simulink model "benchmark_model"  (R2021a)
settings: Solver=ode1  StartTime=0.0  StopTime=Tend  FixedStep=0.0001  MaxStep=0.1  MinStep=0.0001  AbsTol=0.01  EnableMultiTasking=on
undefined symbols (not defined in the file): A1, A2, AL, AM0, AREA, BORE, C_EGR, c_f, c_T, CAIR, cCO, cCO2, cH2, cH2O, cHC, cN2, CO, CO2, cO2, DEN0, DiscIntNeverNeededParam, EGR_dia, EGR_sk, EX_AREA, EX_M_AR, EXO, FD0, FOM, FR0, FR_C1, FR_C2, FR_C3, FR_C4, FR_C5, H2, H2O, HC, INC, INO, KET, Kex, Kh, MAS0, MCh, MHC, MN2, MO2, MOLcylT, N2, O2, PR0, R150, Rabs, SPEC, TBORE, Th_HC, Th_knock, THEX, THIN, TM0 ... (+9)
libraries: pid_lib x1
(part 3 of 6)

== system benchmark_model/ENGINE/engine_s/cylinders/cyl2/cyl/cyl_conc ==
  mol_bs : Inport
  mol_us : Inport  Port=2
  Add : Sum
  Divide : Product  Inputs=*/
  Sum of Elements : Sum  Inputs=+
  cyl_conc : Outport  PortDimensions=7
  mix_mol : Outport  Port=2  PortDimensions=7
  wires:
  Divide/1 -> cyl_conc/1
  mol_bs/1 -> Add/1
  mol_us/1 -> Add/2
  Sum of Elements/1 -> Divide/2
  Add/1 -> mix_mol/1, Divide/1, Sum of Elements/1

== system benchmark_model/ENGINE/engine_s/cylinders/cyl2/cyl/frame ==
  rps : Inport
  rad : Inport  Port=2
  VT : Inport  Port=3
  SA : Inport  Port=4
  tr_inc : Inport  Port=5
  mol_s : Inport  Port=6
  AF : Inport  Port=7
  KL : Inport  Port=8
  EGR : Inport  Port=9
  Init_cyl_gas : Subsystem
  Product : Product  RndMeth=Zero
  Product1 : Product  RndMeth=Zero
  Product2 : Product  RndMeth=Zero
  ratio_burnt1 : Subsystem
  burning gas : Outport
  q : Outport  Port=2
  burnt_gas : Outport  Port=3
  QR : Outport  Port=4
  QA : Outport  Port=5
  af : Outport  Port=6
  Qmax : Outport  Port=7
  wires:
  VT/1 -> ratio_burnt1/7(VT)
  ratio_burnt1/3(Q) -> QA/1
  EGR/1 -> ratio_burnt1/6(EGR)
  ratio_burnt1/2(QR) -> QR/1
  SA/1 -> ratio_burnt1/5(SA)
  KL/1 -> ratio_burnt1/4(KL)
  AF/1 -> ratio_burnt1/3(AF)
  tr_inc/1 -> Init_cyl_gas/1(tr_inc)
  mol_s/1 -> Init_cyl_gas/2(mol_s)
  Init_cyl_gas/4(af) -> af/1
  rad/1 -> ratio_burnt1/2(rad)
  rps/1 -> ratio_burnt1/1(rps)
  ratio_burnt1/1(burnt_ratio) -> Product1/1, Product2/1, Product/1
  Init_cyl_gas/2(Qmax) -> Product1/2, Qmax/1
  Product/1 -> burning gas/1
  Init_cyl_gas/1(init_gas) -> Product/2
  Product1/1 -> q/1
  Product2/1 -> burnt_gas/1
  Init_cyl_gas/3(b_comp) -> Product2/2

== system benchmark_model/ENGINE/engine_s/cylinders/cyl2/cyl/heat_trans ==
  rps : Inport
  pc : Inport  Port=2
  tc : Inport  Port=3
  vol : Inport  Port=4
  Constant5 : Constant  Value=TW0
  Gain : Gain  Gain=Kh
  Product : Product  RndMeth=Zero
  cal_cyl_ar : Subsystem
  cal_qw : Subsystem
  cyl_wall : Subsystem
  qw : Outport
  wires:
  Gain/1 -> qw/1, cyl_wall/1(qw_v)
  cal_cyl_ar/1(cyl_ar) -> Product/1
  vol/1 -> cal_cyl_ar/1(vol)
  Constant5/1 -> cyl_wall/2(Tw0)
  Product/1 -> Gain/1
  cal_qw/1(qw) -> Product/2
  cyl_wall/1(Tw) -> cal_qw/4(Tw)
  tc/1 -> cal_qw/3(Tg)
  rps/1 -> cal_qw/2(rps)
  pc/1 -> cal_qw/1(pc)

== system benchmark_model/ENGINE/engine_s/cylinders/cyl2/cyl/knock_Integral ==
  pc : Inport
  Tc : Inport  Port=2
  Qmax : Inport  Port=3
  rad : Inport  Port=4
  rps : Inport  Port=5
  QA : Inport  Port=6
  Constant : Constant
  Constant1 : Constant  Value=(180-EXO-3)*pi/180
  Constant2 : Constant
  Logical Operator : Logic  Operator=OR  AllPortsSameDT=off  OutDataTypeStr=boolean
  Product : Product
  Relational Operator : RelationalOperator  OutDataTypeStr=boolean  RndMeth=Nearest
  Relational Operator1 : RelationalOperator  OutDataTypeStr=boolean  RndMeth=Nearest
  Subsystem1 : Subsystem
  Switch : Switch  Threshold=0.5
  Triggered Subsystem : Subsystem  TreatAsAtomicUnit=on
  ki : Outport
  ki1 : Outport  Port=2
  wires:
  Triggered Subsystem/1(AI_Q) -> Product/1
  Constant2/1 -> Switch/3
  Switch/1 -> Triggered Subsystem/1(QA_max)
  Logical Operator/1 -> Triggered Subsystem/Trigger
  Relational Operator1/1 -> Logical Operator/2, Switch/2
  Relational Operator/1 -> Logical Operator/1
  QA/1 -> Triggered Subsystem/2(QA), Switch/1
  Qmax/1 -> Product/2
  Product/1 -> ki1/1
  Constant1/1 -> Relational Operator1/2
  Constant/1 -> Relational Operator/2
  Subsystem1/1(ki) -> ki/1, Relational Operator/1
  rad/1 -> Subsystem1/4(rad), Relational Operator1/1
  Tc/1 -> Subsystem1/3(Tc)
  rps/1 -> Subsystem1/2(rps)
  pc/1 -> Subsystem1/1(pc)

== system benchmark_model/ENGINE/engine_s/cylinders/cyl2/cyl/ramining ratio of fuel ==
  rad : Inport
  QA : Inport  Port=2
  Constant1 : Constant  Value=(180-EXO-3)*pi/180
  Memory : Memory
  Relational Operator1 : RelationalOperator  OutDataTypeStr=boolean  RndMeth=Nearest
  Triggered Subsystem : Subsystem  TreatAsAtomicUnit=on
  r_HC : Outport
  wires:
  Memory/1 -> Triggered Subsystem/1(QA)
  Relational Operator1/1 -> Triggered Subsystem/Trigger
  rad/1 -> Relational Operator1/1
  QA/1 -> Memory/1
  Triggered Subsystem/1(AI_Q) -> r_HC/1
  Constant1/1 -> Relational Operator1/2

== system benchmark_model/ENGINE/engine_s/cylinders/cyl2/cyl/unburnt_gass ==
  Nfuel : Inport
  burning : Inport  Port=2
  gas_in : Inport  Port=3
  gas_out : Inport  Port=4
  trig_mix : Inport  Port=5
  mix_mol : Inport  Port=6
  Mass_Int : Integrator  ExternalReset=rising  InitialConditionSource=external  InitialCondition=MAS0
  Memory1 : Memory
  Memory2 : Memory
  Sum : Sum  Inputs=+--  InputSameDT=on  SaturateOnIntegerOverflow=on  OutDataTypeStr=Inherit: Same as first input
  add_fuel1 : Subsystem
  init&trig : Subsystem  mask{NHC=cHC*MOLcylT, NCO2=cCO2*MOLcylT, NCO=cCO*MOLcylT, NO2=cO2*MOLcylT, NH2=cH2*MOLcylT, NH2O=cH2O*MOLcylT, NN2=cN2*MOLcylT}
      mask prompts: NHC "initial HC mol"; NCO2 "initial CO2 mol"; NCO "initial CO mol"; NO2 "initial O2 mol"; NH2 "initial H2 mol"; NH2O "initial H2O mol"; NN2 "initial N2 mol"
  mol_us : Outport  InitialOutput=0
  wires:
  Memory1/1 -> init&trig/2(value)
  trig_mix/1 -> Memory2/1
  Memory2/1 -> Mass_Int/2, init&trig/1(trig)
  add_fuel1/1(add_fuel) -> Sum/1
  Nfuel/1 -> add_fuel1/1(Nfuel)
  gas_in/1 -> add_fuel1/2(mol)
  init&trig/1(init) -> Mass_Int/3
  mix_mol/1 -> Memory1/1
  Mass_Int/1 -> mol_us/1
  burning/1 -> Sum/3
  Sum/1 -> Mass_Int/1
  gas_out/1 -> Sum/2

== system benchmark_model/ENGINE/engine_s/cylinders/cyl2/selectors/Triggered Subsystem1 ==
  sa : Inport
  Trigger : TriggerPort  VariantControl=(inherit)
  req_sa : Outport  InitialOutput=[20]
  wires:
  sa/1 -> req_sa/1

== system benchmark_model/ENGINE/engine_s/cylinders/cyl2/selectors/Triggered Subsystem2 ==
  int_mc : Inport
  Trigger : TriggerPort  VariantControl=(inherit)
  O2_mol : Outport  InitialOutput=[1.0e-19]
  wires:
  int_mc/1 -> O2_mol/1

== system benchmark_model/ENGINE/engine_s/cylinders/cyl2/selectors/Triggered Subsystem3 ==
  int_mc : Inport
  Trigger : TriggerPort  VariantControl=(inherit)
  MC : Outport  InitialOutput=[1.0e-19]
  wires:
  int_mc/1 -> MC/1

== system benchmark_model/ENGINE/engine_s/cylinders/cyl2/selectors/effective_O2_flow ==
  fml : Inport
  Gain : Gain  Gain=1+y/4
  Gain1 : Gain  Gain=0.5
  Gain2 : Gain  Gain=0.5
  Selector : Selector  InputPortWidth=7  IndexOptions=Index vector (dialog)  Indices=[4]  OutputSizes=1
  Selector1 : Selector  InputPortWidth=7  IndexOptions=Index vector (dialog)  Indices=[1]  OutputSizes=1
  Selector2 : Selector  InputPortWidth=7  IndexOptions=Index vector (dialog)  Indices=[3]  OutputSizes=1
  Selector3 : Selector  InputPortWidth=7  IndexOptions=Index vector (dialog)  Indices=[5]  OutputSizes=1
  Subtract : Sum  Inputs=+---
  fO2_mol : Outport
  wires:
  Gain2/1 -> Subtract/4
  Gain1/1 -> Subtract/3
  Selector3/1 -> Gain2/1
  Selector2/1 -> Gain1/1
  Gain/1 -> Subtract/2
  Selector1/1 -> Gain/1
  Selector/1 -> Subtract/1
  fml/1 -> Selector3/1, Selector2/1, Selector1/1, Selector/1
  Subtract/1 -> fO2_mol/1

== system benchmark_model/ENGINE/engine_s/cylinders/cyl2/selectors/fuel_behavior ==
  MC : Inport
  fi : Inport  Port=2
  rps : Inport  Port=3
  Trigger : TriggerPort  VariantControl=(inherit)
  Discrete-Time Integrator : DiscreteIntegrator  SampleTime=-1  ICPrevOutput=DiscIntNeverNeededParam  ICPrevScaledInput=DiscIntNeverNeededParam
  Terminator : Terminator
  Terminator3 : Terminator
  fc : Outport  InitialOutput=[0]
  sum_fc : Outport  Port=2  InitialOutput=[0]
  wires:
  Discrete-Time Integrator/1 -> sum_fc/1
  rps/1 -> Terminator/1
  MC/1 -> Terminator3/1
  fi/1 -> fc/1, Discrete-Time Integrator/1

== system benchmark_model/ENGINE/engine_s/cylinders/cyl2/selectors/selector ==
  st : Inport
  ECU_sa : Inport  Port=2
  ECU_fi : Inport  Port=3
  Saturation : Saturate  UpperLimit=inf  LowerLimit=0
  Selector : Selector  InputPortWidth=4  IndexOptions=Index vector (dialog)  Indices=[2]  OutputSizes=[(-2)]
  Selector2 : Selector  InputPortWidth=4  IndexOptions=Index vector (dialog)  Indices=[2]  OutputSizes=[(-2)]
  mod720(u,4*pi) : Subsystem
  rad : Outport
  sa : Outport  Port=2
  fi : Outport  Port=3
  wires:
  Selector2/1 -> sa/1
  ECU_fi/1 -> Saturation/1
  ECU_sa/1 -> Selector2/1
  st/1 -> Selector/1
  mod720(u,4*pi)/1(y) -> rad/1
  Saturation/1 -> fi/1
  Selector/1 -> mod720(u,4*pi)/1(u)

== system benchmark_model/ENGINE/engine_s/cylinders/cyl2/selectors/trig_MC ==
  deg : Inport
  ECU_vvt : Inport  Port=2
  Constant : Constant  Value=541+INC
  Gain : Gain  Gain=180/pi
  Relational Operator : RelationalOperator  OutDataTypeStr=boolean  RndMeth=Nearest
  Subtract : Sum
  flg_inc : Outport
  wires:
  Gain/1 -> Subtract/1
  Constant/1 -> Subtract/2
  ECU_vvt/1 -> Gain/1
  Subtract/1 -> Relational Operator/2
  Relational Operator/1 -> flg_inc/1
  deg/1 -> Relational Operator/1

== system benchmark_model/ENGINE/engine_s/cylinders/cyl2/selectors/trig_fi ==
  deg : Inport
  Constant : Constant  Value=361
  Relational Operator : RelationalOperator  OutDataTypeStr=boolean  RndMeth=Nearest
  flg_fi : Outport
  wires:
  Relational Operator/1 -> flg_fi/1
  deg/1 -> Relational Operator/1
  Constant/1 -> Relational Operator/2

== system benchmark_model/ENGINE/engine_s/cylinders/cyl2/selectors/trig_fi1 ==
  deg : Inport
  ECU_vvt : Inport  Port=2
  Constant : Constant  Value=360-INO-1
  Gain : Gain  Gain=180/pi
  Relational Operator : RelationalOperator  OutDataTypeStr=boolean  RndMeth=Nearest
  Subtract : Sum
  flg_fi : Outport
  wires:
  Constant/1 -> Subtract/2
  Subtract/1 -> Relational Operator/2
  Gain/1 -> Subtract/1
  ECU_vvt/1 -> Gain/1
  deg/1 -> Relational Operator/1
  Relational Operator/1 -> flg_fi/1

== system benchmark_model/ENGINE/engine_s/cylinders/cyl3/cyl/Energy_Int ==
  p : Inport
  qw : Inport  Port=2
  e_out : Inport  Port=3
  e_in : Inport  Port=4
  rad : Inport  Port=5
  rps : Inport  Port=6
  q : Inport  Port=7
  Constant : Constant  Value=PR0
  Product : Product  RndMeth=Zero
  Product1 : Product  RndMeth=Zero
  Subtract : Sum  Inputs=+-
  Sum2 : Sum  Inputs=+--+-  InputSameDT=on  SaturateOnIntegerOverflow=on  OutDataTypeStr=Inherit: Same as first input
  dvol : Subsystem
  int_e : Integrator  InitialCondition=(FD0/2.0)*PR0*VT
  int_pdv : Integrator
  E_mech : Outport  InitialOutput=0
  E : Outport  Port=2  InitialOutput=0
  wires:
  qw/1 -> Sum2/2
  e_out/1 -> Sum2/3
  Product/1 -> Sum2/5
  e_in/1 -> Sum2/4
  q/1 -> Sum2/1
  int_e/1 -> E/1
  Sum2/1 -> int_e/1
  rad/1 -> dvol/1(rad)
  dvol/1(dvol) -> Product1/1, Product/2
  rps/1 -> dvol/2(rps)
  int_pdv/1 -> E_mech/1
  p/1 -> Subtract/1, Product/1
  Constant/1 -> Subtract/2
  Subtract/1 -> Product1/2
  Product1/1 -> int_pdv/1

== system benchmark_model/ENGINE/engine_s/cylinders/cyl3/cyl/burnt_gass ==
  gas_in : Inport
  tr_mix : Inport  Port=2
  Mass_Int : Integrator  ExternalReset=rising  InitialCondition=[0;0;0;0;0;0;0]
  Memory2 : Memory
  mol_bs : Outport  PortDimensions=7  InitialOutput=0
  wires:
  Mass_Int/1 -> mol_bs/1
  gas_in/1 -> Mass_Int/1
  tr_mix/1 -> Memory2/1
  Memory2/1 -> Mass_Int/2

== system benchmark_model/ENGINE/engine_s/cylinders/cyl3/cyl/cal_cyl_state ==
  E : Inport
  mol_u : Inport  Port=2
  mol_b : Inport  Port=3
  rad : Inport  Port=4
  Add2 : Sum
  Constant : Constant  Value=SPEC
  Dot Product2 : DotProduct  InputSameDT=on  OutDataTypeStr=Inherit: Inherit via internal rule
  Dot Product3 : DotProduct  InputSameDT=on  OutDataTypeStr=Inherit: Inherit via internal rule
  Sum of Elements : Sum  Inputs=+
  cal_state : Subsystem
  cyl_vol : MATLAB Function  TreatAsAtomicUnit=on
  freedom : Constant  Value=FOM
  weight_mol : Constant  Value=WOM
  pc : Outport  InitialOutput=0
  tc : Outport  Port=2  InitialOutput=0
  vol : Outport  Port=3  InitialOutput=0
  cyl_st : Outport  Port=4  InitialOutput=0
  wires:
  E/1 -> cal_state/4(E)
  rad/1 -> cyl_vol/1(u)
  Constant/1 -> cyl_vol/2(SPEC)
  cal_state/1(pc) -> pc/1
  cal_state/2(tc) -> tc/1
  cal_state/3(cyl_st) -> cyl_st/1
  cyl_vol/1(vol) -> vol/1, cal_state/5(vol)
  weight_mol/1 -> Dot Product2/1
  mol_b/1 -> Add2/1
  mol_u/1 -> Add2/2
  Add2/1 -> Sum of Elements/1, Dot Product2/2, Dot Product3/1
  freedom/1 -> Dot Product3/2
  Sum of Elements/1 -> cal_state/2(n)
  Dot Product2/1 -> cal_state/1(m)
  Dot Product3/1 -> cal_state/3(f)

== system benchmark_model/ENGINE/engine_s/cylinders/cyl3/cyl/cal_torque ==
  E_mech : Inport
  Trigger : TriggerPort  VariantControl=(inherit)  PortDimensions=1
  Constant : Constant  Value=4*pi
  Divide : Product  Inputs=*/
  Subtract : Sum  Inputs=+-
  Unit Delay : UnitDelay  SampleTime=-1  HasFrameUpgradeWarning=on
  Torque : Outport
  wires:
  Unit Delay/1 -> Subtract/2
  E_mech/1 -> Subtract/1, Unit Delay/1
  Subtract/1 -> Divide/1
  Divide/1 -> Torque/1
  Constant/1 -> Divide/2

== system benchmark_model/ENGINE/engine_s/cylinders/cyl3/cyl/crank ==
  ecu : Inport
  Constant : Constant  Value=(180-EXO-1)*pi/180
  Constant2 : Constant  Value=(540+INC)*pi/180
  Relational Operator : RelationalOperator  OutDataTypeStr=boolean  RndMeth=Nearest
  Relational Operator2 : RelationalOperator  OutDataTypeStr=boolean  RndMeth=Nearest
  Selector : Selector  InputPortWidth=6  IndexOptions=Index vector (dialog)  Indices=1  OutputSizes=[(-2)]
  Selector1 : Selector  InputPortWidth=6  IndexOptions=Index vector (dialog)  Indices=[3]  OutputSizes=[(-2)]
  Selector2 : Selector  InputPortWidth=6  IndexOptions=Index vector (dialog)  Indices=[5]  OutputSizes=[(-2)]
  Selector3 : Selector  InputPortWidth=6  IndexOptions=Index vector (dialog)  Indices=2  OutputSizes=[(-2)]
  Selector4 : Selector  InputPortWidth=6  IndexOptions=Index vector (dialog)  Indices=6  OutputSizes=[(-2)]
  Selector5 : Selector  InputPortWidth=6  IndexOptions=Index vector (dialog)  Indices=6  OutputSizes=[(-2)]
  Subsystem1 : Subsystem
  Subtract : Sum  Inputs=+++
  inj_start : Subsystem
  mol_flow_rate : Subsystem
  trig_mix : Outport  PortDimensions=1
  rad : Outport  Port=2
  tr_inc : Outport  Port=3  PortDimensions=1
  SA : Outport  Port=4
  VT : Outport  Port=5
  Nfuel : Outport  Port=6
  wires:
  Selector/1 -> inj_start/1(rad), rad/1, Relational Operator2/1, Relational Operator/1
  Constant/1 -> Relational Operator/2
  ecu/1 -> Selector5/1, Selector4/1, Selector/1, Selector3/1, Selector2/1, Selector1/1
  Selector2/1 -> mol_flow_rate/1(rps)  "rps"
  Relational Operator2/1 -> tr_inc/1
  Selector3/1 -> SA/1
  Subtract/1 -> Relational Operator2/2
  Selector5/1 -> Subtract/1, VT/1
  Selector4/1 -> Subtract/3
  Constant2/1 -> Subtract/2
  Relational Operator/1 -> trig_mix/1
  inj_start/1(trig_inj) -> Subsystem1/1(trig_inj)
  Selector1/1 -> Subsystem1/2(fc)
  mol_flow_rate/1(N/s) -> Subsystem1/3(N/s)
  Subsystem1/1(N_fuel) -> Nfuel/1

== system benchmark_model/ENGINE/engine_s/cylinders/cyl3/cyl/cyl_conc ==
  mol_bs : Inport
  mol_us : Inport  Port=2
  Add : Sum
  Divide : Product  Inputs=*/
  Sum of Elements : Sum  Inputs=+
  cyl_conc : Outport  PortDimensions=7
  mix_mol : Outport  Port=2  PortDimensions=7
  wires:
  Add/1 -> Sum of Elements/1, Divide/1, mix_mol/1
  Sum of Elements/1 -> Divide/2
  mol_us/1 -> Add/2
  mol_bs/1 -> Add/1
  Divide/1 -> cyl_conc/1

== system benchmark_model/ENGINE/engine_s/cylinders/cyl3/cyl/frame ==
  rps : Inport
  rad : Inport  Port=2
  VT : Inport  Port=3
  SA : Inport  Port=4
  tr_inc : Inport  Port=5
  mol_s : Inport  Port=6
  AF : Inport  Port=7
  KL : Inport  Port=8
  EGR : Inport  Port=9
  Init_cyl_gas : Subsystem
  Product : Product  RndMeth=Zero
  Product1 : Product  RndMeth=Zero
  Product2 : Product  RndMeth=Zero
  ratio_burnt1 : Subsystem
  burning gas : Outport
  q : Outport  Port=2
  burnt_gas : Outport  Port=3
  QR : Outport  Port=4
  QA : Outport  Port=5
  af : Outport  Port=6
  Qmax : Outport  Port=7
  wires:
  Init_cyl_gas/3(b_comp) -> Product2/2
  Product2/1 -> burnt_gas/1
  Product1/1 -> q/1
  Init_cyl_gas/1(init_gas) -> Product/2
  Product/1 -> burning gas/1
  Init_cyl_gas/2(Qmax) -> Qmax/1, Product1/2
  ratio_burnt1/1(burnt_ratio) -> Product/1, Product2/1, Product1/1
  rps/1 -> ratio_burnt1/1(rps)
  rad/1 -> ratio_burnt1/2(rad)
  Init_cyl_gas/4(af) -> af/1
  mol_s/1 -> Init_cyl_gas/2(mol_s)
  tr_inc/1 -> Init_cyl_gas/1(tr_inc)
  AF/1 -> ratio_burnt1/3(AF)
  KL/1 -> ratio_burnt1/4(KL)
  SA/1 -> ratio_burnt1/5(SA)
  ratio_burnt1/2(QR) -> QR/1
  EGR/1 -> ratio_burnt1/6(EGR)
  ratio_burnt1/3(Q) -> QA/1
  VT/1 -> ratio_burnt1/7(VT)

== system benchmark_model/ENGINE/engine_s/cylinders/cyl3/cyl/heat_trans ==
  rps : Inport
  pc : Inport  Port=2
  tc : Inport  Port=3
  vol : Inport  Port=4
  Constant5 : Constant  Value=TW0
  Gain : Gain  Gain=Kh
  Product : Product  RndMeth=Zero
  cal_cyl_ar : Subsystem
  cal_qw : Subsystem
  cyl_wall : Subsystem
  qw : Outport
  wires:
  pc/1 -> cal_qw/1(pc)
  rps/1 -> cal_qw/2(rps)
  tc/1 -> cal_qw/3(Tg)
  cyl_wall/1(Tw) -> cal_qw/4(Tw)
  cal_qw/1(qw) -> Product/2
  Product/1 -> Gain/1
  Constant5/1 -> cyl_wall/2(Tw0)
  vol/1 -> cal_cyl_ar/1(vol)
  cal_cyl_ar/1(cyl_ar) -> Product/1
  Gain/1 -> cyl_wall/1(qw_v), qw/1

== system benchmark_model/ENGINE/engine_s/cylinders/cyl3/cyl/knock_Integral ==
  pc : Inport
  Tc : Inport  Port=2
  Qmax : Inport  Port=3
  rad : Inport  Port=4
  rps : Inport  Port=5
  QA : Inport  Port=6
  Constant : Constant
  Constant1 : Constant  Value=(180-EXO-3)*pi/180
  Constant2 : Constant
  Logical Operator : Logic  Operator=OR  AllPortsSameDT=off  OutDataTypeStr=boolean
  Product : Product
  Relational Operator : RelationalOperator  OutDataTypeStr=boolean  RndMeth=Nearest
  Relational Operator1 : RelationalOperator  OutDataTypeStr=boolean  RndMeth=Nearest
  Subsystem1 : Subsystem
  Switch : Switch  Threshold=0.5
  Triggered Subsystem : Subsystem  TreatAsAtomicUnit=on
  ki : Outport
  ki1 : Outport  Port=2
  wires:
  pc/1 -> Subsystem1/1(pc)
  rps/1 -> Subsystem1/2(rps)
  Tc/1 -> Subsystem1/3(Tc)
  rad/1 -> Relational Operator1/1, Subsystem1/4(rad)
  Subsystem1/1(ki) -> Relational Operator/1, ki/1
  Constant/1 -> Relational Operator/2
  Constant1/1 -> Relational Operator1/2
  Product/1 -> ki1/1
  Qmax/1 -> Product/2
  QA/1 -> Switch/1, Triggered Subsystem/2(QA)
  Relational Operator/1 -> Logical Operator/1
  Relational Operator1/1 -> Switch/2, Logical Operator/2
  Logical Operator/1 -> Triggered Subsystem/Trigger
  Switch/1 -> Triggered Subsystem/1(QA_max)
  Constant2/1 -> Switch/3
  Triggered Subsystem/1(AI_Q) -> Product/1

== system benchmark_model/ENGINE/engine_s/cylinders/cyl3/cyl/ramining ratio of fuel ==
  rad : Inport
  QA : Inport  Port=2
  Constant1 : Constant  Value=(180-EXO-3)*pi/180
  Memory : Memory
  Relational Operator1 : RelationalOperator  OutDataTypeStr=boolean  RndMeth=Nearest
  Triggered Subsystem : Subsystem  TreatAsAtomicUnit=on
  r_HC : Outport
  wires:
  Constant1/1 -> Relational Operator1/2
  Triggered Subsystem/1(AI_Q) -> r_HC/1
  QA/1 -> Memory/1
  rad/1 -> Relational Operator1/1
  Relational Operator1/1 -> Triggered Subsystem/Trigger
  Memory/1 -> Triggered Subsystem/1(QA)

== system benchmark_model/ENGINE/engine_s/cylinders/cyl3/cyl/unburnt_gass ==
  Nfuel : Inport
  burning : Inport  Port=2
  gas_in : Inport  Port=3
  gas_out : Inport  Port=4
  trig_mix : Inport  Port=5
  mix_mol : Inport  Port=6
  Mass_Int : Integrator  ExternalReset=rising  InitialConditionSource=external  InitialCondition=MAS0
  Memory1 : Memory
  Memory2 : Memory
  Sum : Sum  Inputs=+--  InputSameDT=on  SaturateOnIntegerOverflow=on  OutDataTypeStr=Inherit: Same as first input
  add_fuel1 : Subsystem
  init&trig : Subsystem  mask{NHC=cHC*MOLcylT, NCO2=cCO2*MOLcylT, NCO=cCO*MOLcylT, NO2=cO2*MOLcylT, NH2=cH2*MOLcylT, NH2O=cH2O*MOLcylT, NN2=cN2*MOLcylT}
      mask prompts: NHC "initial HC mol"; NCO2 "initial CO2 mol"; NCO "initial CO mol"; NO2 "initial O2 mol"; NH2 "initial H2 mol"; NH2O "initial H2O mol"; NN2 "initial N2 mol"
  mol_us : Outport  InitialOutput=0
  wires:
  gas_out/1 -> Sum/2
  Sum/1 -> Mass_Int/1
  burning/1 -> Sum/3
  Mass_Int/1 -> mol_us/1
  mix_mol/1 -> Memory1/1
  init&trig/1(init) -> Mass_Int/3
  gas_in/1 -> add_fuel1/2(mol)
  Nfuel/1 -> add_fuel1/1(Nfuel)
  add_fuel1/1(add_fuel) -> Sum/1
  Memory2/1 -> init&trig/1(trig), Mass_Int/2
  trig_mix/1 -> Memory2/1
  Memory1/1 -> init&trig/2(value)

== system benchmark_model/ENGINE/engine_s/cylinders/cyl3/selectors/Triggered Subsystem1 ==
  sa : Inport
  Trigger : TriggerPort  VariantControl=(inherit)
  req_sa : Outport  InitialOutput=[20]
  wires:
  sa/1 -> req_sa/1

== system benchmark_model/ENGINE/engine_s/cylinders/cyl3/selectors/Triggered Subsystem2 ==
  int_mc : Inport
  Trigger : TriggerPort  VariantControl=(inherit)
  O2_mol : Outport  InitialOutput=[1.0e-19]
  wires:
  int_mc/1 -> O2_mol/1

== system benchmark_model/ENGINE/engine_s/cylinders/cyl3/selectors/Triggered Subsystem3 ==
  int_mc : Inport
  Trigger : TriggerPort  VariantControl=(inherit)
  MC : Outport  InitialOutput=[1.0e-19]
  wires:
  int_mc/1 -> MC/1

== system benchmark_model/ENGINE/engine_s/cylinders/cyl3/selectors/effective_O2_flow ==
  fml : Inport
  Gain : Gain  Gain=1+y/4
  Gain1 : Gain  Gain=0.5
  Gain2 : Gain  Gain=0.5
  Selector : Selector  InputPortWidth=7  IndexOptions=Index vector (dialog)  Indices=[4]  OutputSizes=1
  Selector1 : Selector  InputPortWidth=7  IndexOptions=Index vector (dialog)  Indices=[1]  OutputSizes=1
  Selector2 : Selector  InputPortWidth=7  IndexOptions=Index vector (dialog)  Indices=[3]  OutputSizes=1
  Selector3 : Selector  InputPortWidth=7  IndexOptions=Index vector (dialog)  Indices=[5]  OutputSizes=1
  Subtract : Sum  Inputs=+---
  fO2_mol : Outport
  wires:
  Subtract/1 -> fO2_mol/1
  fml/1 -> Selector/1, Selector1/1, Selector2/1, Selector3/1
  Selector/1 -> Subtract/1
  Selector1/1 -> Gain/1
  Gain/1 -> Subtract/2
  Selector2/1 -> Gain1/1
  Selector3/1 -> Gain2/1
  Gain1/1 -> Subtract/3
  Gain2/1 -> Subtract/4

== system benchmark_model/ENGINE/engine_s/cylinders/cyl3/selectors/fuel_behavior ==
  MC : Inport
  fi : Inport  Port=2
  rps : Inport  Port=3
  Trigger : TriggerPort  VariantControl=(inherit)
  Discrete-Time Integrator : DiscreteIntegrator  SampleTime=-1  ICPrevOutput=DiscIntNeverNeededParam  ICPrevScaledInput=DiscIntNeverNeededParam
  Terminator : Terminator
  Terminator3 : Terminator
  fc : Outport  InitialOutput=[0]
  sum_fc : Outport  Port=2  InitialOutput=[0]
  wires:
  fi/1 -> Discrete-Time Integrator/1, fc/1
  MC/1 -> Terminator3/1
  rps/1 -> Terminator/1
  Discrete-Time Integrator/1 -> sum_fc/1

== system benchmark_model/ENGINE/engine_s/cylinders/cyl3/selectors/selector ==
  st : Inport
  ECU_sa : Inport  Port=2
  ECU_fi : Inport  Port=3
  Saturation : Saturate  UpperLimit=inf  LowerLimit=0
  Selector : Selector  InputPortWidth=4  IndexOptions=Index vector (dialog)  Indices=[3]  OutputSizes=[(-2)]
  Selector2 : Selector  InputPortWidth=4  IndexOptions=Index vector (dialog)  Indices=[3]  OutputSizes=[(-2)]
  mod720(u,4*pi) : Subsystem
  rad : Outport
  sa : Outport  Port=2
  fi : Outport  Port=3
  wires:
  Selector/1 -> mod720(u,4*pi)/1(u)
  Saturation/1 -> fi/1
  mod720(u,4*pi)/1(y) -> rad/1
  st/1 -> Selector/1
  ECU_sa/1 -> Selector2/1
  ECU_fi/1 -> Saturation/1
  Selector2/1 -> sa/1

== system benchmark_model/ENGINE/engine_s/cylinders/cyl3/selectors/trig_MC ==
  deg : Inport
  ECU_vvt : Inport  Port=2
  Constant : Constant  Value=541+INC
  Gain : Gain  Gain=180/pi
  Relational Operator : RelationalOperator  OutDataTypeStr=boolean  RndMeth=Nearest
  Subtract : Sum
  flg_inc : Outport
  wires:
  deg/1 -> Relational Operator/1
  Relational Operator/1 -> flg_inc/1
  Subtract/1 -> Relational Operator/2
  ECU_vvt/1 -> Gain/1
  Constant/1 -> Subtract/2
  Gain/1 -> Subtract/1

== system benchmark_model/ENGINE/engine_s/cylinders/cyl3/selectors/trig_fi ==
  deg : Inport
  Constant : Constant  Value=361
  Relational Operator : RelationalOperator  OutDataTypeStr=boolean  RndMeth=Nearest
  flg_fi : Outport
  wires:
  Constant/1 -> Relational Operator/2
  deg/1 -> Relational Operator/1
  Relational Operator/1 -> flg_fi/1

== system benchmark_model/ENGINE/engine_s/cylinders/cyl3/selectors/trig_fi1 ==
  deg : Inport
  ECU_vvt : Inport  Port=2
  Constant : Constant  Value=360-INO-1
  Gain : Gain  Gain=180/pi
  Relational Operator : RelationalOperator  OutDataTypeStr=boolean  RndMeth=Nearest
  Subtract : Sum
  flg_fi : Outport
  wires:
  Relational Operator/1 -> flg_fi/1
  deg/1 -> Relational Operator/1
  ECU_vvt/1 -> Gain/1
  Gain/1 -> Subtract/1
  Subtract/1 -> Relational Operator/2
  Constant/1 -> Subtract/2

== system benchmark_model/ENGINE/engine_s/cylinders/cyl4/cyl/Energy_Int ==
  p : Inport
  qw : Inport  Port=2
  e_out : Inport  Port=3
  e_in : Inport  Port=4
  rad : Inport  Port=5
  rps : Inport  Port=6
  q : Inport  Port=7
  Constant : Constant  Value=PR0
  Product : Product  RndMeth=Zero
  Product1 : Product  RndMeth=Zero
  Subtract : Sum  Inputs=+-
  Sum2 : Sum  Inputs=+--+-  InputSameDT=on  SaturateOnIntegerOverflow=on  OutDataTypeStr=Inherit: Same as first input
  dvol : Subsystem
  int_e : Integrator  InitialCondition=(FD0/2.0)*PR0*VT
  int_pdv : Integrator
  E_mech : Outport  InitialOutput=0
  E : Outport  Port=2  InitialOutput=0
  wires:
  Product1/1 -> int_pdv/1
  Subtract/1 -> Product1/2
  Constant/1 -> Subtract/2
  p/1 -> Product/1, Subtract/1
  int_pdv/1 -> E_mech/1
  rps/1 -> dvol/2(rps)
  dvol/1(dvol) -> Product/2, Product1/1
  rad/1 -> dvol/1(rad)
  Sum2/1 -> int_e/1
  int_e/1 -> E/1
  q/1 -> Sum2/1
  e_in/1 -> Sum2/4
  Product/1 -> Sum2/5
  e_out/1 -> Sum2/3
  qw/1 -> Sum2/2

== system benchmark_model/ENGINE/engine_s/cylinders/cyl4/cyl/burnt_gass ==
  gas_in : Inport
  tr_mix : Inport  Port=2
  Mass_Int : Integrator  ExternalReset=rising  InitialCondition=[0;0;0;0;0;0;0]
  Memory2 : Memory
  mol_bs : Outport  PortDimensions=7  InitialOutput=0
  wires:
  Memory2/1 -> Mass_Int/2
  tr_mix/1 -> Memory2/1
  gas_in/1 -> Mass_Int/1
  Mass_Int/1 -> mol_bs/1

== system benchmark_model/ENGINE/engine_s/cylinders/cyl4/cyl/cal_cyl_state ==
  E : Inport
  mol_u : Inport  Port=2
  mol_b : Inport  Port=3
  rad : Inport  Port=4
  Add2 : Sum
  Constant : Constant  Value=SPEC
  Dot Product2 : DotProduct  InputSameDT=on  OutDataTypeStr=Inherit: Inherit via internal rule
  Dot Product3 : DotProduct  InputSameDT=on  OutDataTypeStr=Inherit: Inherit via internal rule
  Sum of Elements : Sum  Inputs=+
  cal_state : Subsystem
  cyl_vol : MATLAB Function  TreatAsAtomicUnit=on
  freedom : Constant  Value=FOM
  weight_mol : Constant  Value=WOM
  pc : Outport  InitialOutput=0
  tc : Outport  Port=2  InitialOutput=0
  vol : Outport  Port=3  InitialOutput=0
  cyl_st : Outport  Port=4  InitialOutput=0
  wires:
  Dot Product3/1 -> cal_state/3(f)
  Dot Product2/1 -> cal_state/1(m)
  Sum of Elements/1 -> cal_state/2(n)
  freedom/1 -> Dot Product3/2
  Add2/1 -> Dot Product3/1, Dot Product2/2, Sum of Elements/1
  mol_u/1 -> Add2/2
  mol_b/1 -> Add2/1
  weight_mol/1 -> Dot Product2/1
  cyl_vol/1(vol) -> cal_state/5(vol), vol/1
  cal_state/3(cyl_st) -> cyl_st/1
  cal_state/2(tc) -> tc/1
  cal_state/1(pc) -> pc/1
  Constant/1 -> cyl_vol/2(SPEC)
  rad/1 -> cyl_vol/1(u)
  E/1 -> cal_state/4(E)

== system benchmark_model/ENGINE/engine_s/cylinders/cyl4/cyl/cal_torque ==
  E_mech : Inport
  Trigger : TriggerPort  VariantControl=(inherit)  PortDimensions=1
  Constant : Constant  Value=4*pi
  Divide : Product  Inputs=*/
  Subtract : Sum  Inputs=+-
  Unit Delay : UnitDelay  SampleTime=-1  HasFrameUpgradeWarning=on
  Torque : Outport
  wires:
  Constant/1 -> Divide/2
  Divide/1 -> Torque/1
  Subtract/1 -> Divide/1
  E_mech/1 -> Unit Delay/1, Subtract/1
  Unit Delay/1 -> Subtract/2

== system benchmark_model/ENGINE/engine_s/cylinders/cyl4/cyl/crank ==
  ecu : Inport
  Constant : Constant  Value=(180-EXO-1)*pi/180
  Constant2 : Constant  Value=(540+INC)*pi/180
  Relational Operator : RelationalOperator  OutDataTypeStr=boolean  RndMeth=Nearest
  Relational Operator2 : RelationalOperator  OutDataTypeStr=boolean  RndMeth=Nearest
  Selector : Selector  InputPortWidth=6  IndexOptions=Index vector (dialog)  Indices=1  OutputSizes=[(-2)]
  Selector1 : Selector  InputPortWidth=6  IndexOptions=Index vector (dialog)  Indices=[3]  OutputSizes=[(-2)]
  Selector2 : Selector  InputPortWidth=6  IndexOptions=Index vector (dialog)  Indices=[5]  OutputSizes=[(-2)]
  Selector3 : Selector  InputPortWidth=6  IndexOptions=Index vector (dialog)  Indices=2  OutputSizes=[(-2)]
  Selector4 : Selector  InputPortWidth=6  IndexOptions=Index vector (dialog)  Indices=6  OutputSizes=[(-2)]
  Selector5 : Selector  InputPortWidth=6  IndexOptions=Index vector (dialog)  Indices=6  OutputSizes=[(-2)]
  Subsystem1 : Subsystem
  Subtract : Sum  Inputs=+++
  inj_start : Subsystem
  mol_flow_rate : Subsystem
  trig_mix : Outport  PortDimensions=1
  rad : Outport  Port=2
  tr_inc : Outport  Port=3  PortDimensions=1
  SA : Outport  Port=4
  VT : Outport  Port=5
  Nfuel : Outport  Port=6
  wires:
  Subsystem1/1(N_fuel) -> Nfuel/1
  mol_flow_rate/1(N/s) -> Subsystem1/3(N/s)
  Selector1/1 -> Subsystem1/2(fc)
  inj_start/1(trig_inj) -> Subsystem1/1(trig_inj)
  Relational Operator/1 -> trig_mix/1
  Constant2/1 -> Subtract/2
  Selector4/1 -> Subtract/3
  Selector5/1 -> VT/1, Subtract/1
  Subtract/1 -> Relational Operator2/2
  Selector3/1 -> SA/1
  Relational Operator2/1 -> tr_inc/1
  Selector2/1 -> mol_flow_rate/1(rps)  "rps"
  ecu/1 -> Selector1/1, Selector2/1, Selector3/1, Selector/1, Selector4/1, Selector5/1
  Constant/1 -> Relational Operator/2
  Selector/1 -> Relational Operator/1, Relational Operator2/1, rad/1, inj_start/1(rad)

== system benchmark_model/ENGINE/engine_s/cylinders/cyl4/cyl/cyl_conc ==
  mol_bs : Inport
  mol_us : Inport  Port=2
  Add : Sum
  Divide : Product  Inputs=*/
  Sum of Elements : Sum  Inputs=+
  cyl_conc : Outport  PortDimensions=7
  mix_mol : Outport  Port=2  PortDimensions=7
  wires:
  Divide/1 -> cyl_conc/1
  mol_bs/1 -> Add/1
  mol_us/1 -> Add/2
  Sum of Elements/1 -> Divide/2
  Add/1 -> mix_mol/1, Divide/1, Sum of Elements/1

== system benchmark_model/ENGINE/engine_s/cylinders/cyl4/cyl/frame ==
  rps : Inport
  rad : Inport  Port=2
  VT : Inport  Port=3
  SA : Inport  Port=4
  tr_inc : Inport  Port=5
  mol_s : Inport  Port=6
  AF : Inport  Port=7
  KL : Inport  Port=8
  EGR : Inport  Port=9
  Init_cyl_gas : Subsystem
  Product : Product  RndMeth=Zero
  Product1 : Product  RndMeth=Zero
  Product2 : Product  RndMeth=Zero
  ratio_burnt1 : Subsystem
  burning gas : Outport
  q : Outport  Port=2
  burnt_gas : Outport  Port=3
  QR : Outport  Port=4
  QA : Outport  Port=5
  af : Outport  Port=6
  Qmax : Outport  Port=7
  wires:
  VT/1 -> ratio_burnt1/7(VT)
  ratio_burnt1/3(Q) -> QA/1
  EGR/1 -> ratio_burnt1/6(EGR)
  ratio_burnt1/2(QR) -> QR/1
  SA/1 -> ratio_burnt1/5(SA)
  KL/1 -> ratio_burnt1/4(KL)
  AF/1 -> ratio_burnt1/3(AF)
  tr_inc/1 -> Init_cyl_gas/1(tr_inc)
  mol_s/1 -> Init_cyl_gas/2(mol_s)
  Init_cyl_gas/4(af) -> af/1
  rad/1 -> ratio_burnt1/2(rad)
  rps/1 -> ratio_burnt1/1(rps)
  ratio_burnt1/1(burnt_ratio) -> Product1/1, Product2/1, Product/1
  Init_cyl_gas/2(Qmax) -> Product1/2, Qmax/1
  Product/1 -> burning gas/1
  Init_cyl_gas/1(init_gas) -> Product/2
  Product1/1 -> q/1
  Product2/1 -> burnt_gas/1
  Init_cyl_gas/3(b_comp) -> Product2/2

== system benchmark_model/ENGINE/engine_s/cylinders/cyl4/cyl/heat_trans ==
  rps : Inport
  pc : Inport  Port=2
  tc : Inport  Port=3
  vol : Inport  Port=4
  Constant5 : Constant  Value=TW0
  Gain : Gain  Gain=Kh
  Product : Product  RndMeth=Zero
  cal_cyl_ar : Subsystem
  cal_qw : Subsystem
  cyl_wall : Subsystem
  qw : Outport
  wires:
  Gain/1 -> qw/1, cyl_wall/1(qw_v)
  cal_cyl_ar/1(cyl_ar) -> Product/1
  vol/1 -> cal_cyl_ar/1(vol)
  Constant5/1 -> cyl_wall/2(Tw0)
  Product/1 -> Gain/1
  cal_qw/1(qw) -> Product/2
  cyl_wall/1(Tw) -> cal_qw/4(Tw)
  tc/1 -> cal_qw/3(Tg)
  rps/1 -> cal_qw/2(rps)
  pc/1 -> cal_qw/1(pc)

== system benchmark_model/ENGINE/engine_s/cylinders/cyl4/cyl/knock_Integral ==
  pc : Inport
  Tc : Inport  Port=2
  Qmax : Inport  Port=3
  rad : Inport  Port=4
  rps : Inport  Port=5
  QA : Inport  Port=6
  Constant : Constant
  Constant1 : Constant  Value=(180-EXO-3)*pi/180
  Constant2 : Constant
  Logical Operator : Logic  Operator=OR  AllPortsSameDT=off  OutDataTypeStr=boolean
  Product : Product
  Relational Operator : RelationalOperator  OutDataTypeStr=boolean  RndMeth=Nearest
  Relational Operator1 : RelationalOperator  OutDataTypeStr=boolean  RndMeth=Nearest
  Subsystem1 : Subsystem
  Switch : Switch  Threshold=0.5
  Triggered Subsystem : Subsystem  TreatAsAtomicUnit=on
  ki : Outport
  ki1 : Outport  Port=2
  wires:
  Triggered Subsystem/1(AI_Q) -> Product/1
  Constant2/1 -> Switch/3
  Switch/1 -> Triggered Subsystem/1(QA_max)
  Logical Operator/1 -> Triggered Subsystem/Trigger
  Relational Operator1/1 -> Logical Operator/2, Switch/2
  Relational Operator/1 -> Logical Operator/1
  QA/1 -> Triggered Subsystem/2(QA), Switch/1
  Qmax/1 -> Product/2
  Product/1 -> ki1/1
  Constant1/1 -> Relational Operator1/2
  Constant/1 -> Relational Operator/2
  Subsystem1/1(ki) -> ki/1, Relational Operator/1
  rad/1 -> Subsystem1/4(rad), Relational Operator1/1
  Tc/1 -> Subsystem1/3(Tc)
  rps/1 -> Subsystem1/2(rps)
  pc/1 -> Subsystem1/1(pc)

== system benchmark_model/ENGINE/engine_s/cylinders/cyl4/cyl/ramining ratio of fuel ==
  rad : Inport
  QA : Inport  Port=2
  Constant1 : Constant  Value=(180-EXO-3)*pi/180
  Memory : Memory
  Relational Operator1 : RelationalOperator  OutDataTypeStr=boolean  RndMeth=Nearest
  Triggered Subsystem : Subsystem  TreatAsAtomicUnit=on
  r_HC : Outport
  wires:
  Memory/1 -> Triggered Subsystem/1(QA)
  Relational Operator1/1 -> Triggered Subsystem/Trigger
  rad/1 -> Relational Operator1/1
  QA/1 -> Memory/1
  Triggered Subsystem/1(AI_Q) -> r_HC/1
  Constant1/1 -> Relational Operator1/2

== system benchmark_model/ENGINE/engine_s/cylinders/cyl4/cyl/unburnt_gass ==
  Nfuel : Inport
  burning : Inport  Port=2
  gas_in : Inport  Port=3
  gas_out : Inport  Port=4
  trig_mix : Inport  Port=5
  mix_mol : Inport  Port=6
  Mass_Int : Integrator  ExternalReset=rising  InitialConditionSource=external  InitialCondition=MAS0
  Memory1 : Memory
  Memory2 : Memory
  Sum : Sum  Inputs=+--  InputSameDT=on  SaturateOnIntegerOverflow=on  OutDataTypeStr=Inherit: Same as first input
  add_fuel1 : Subsystem
  init&trig : Subsystem  mask{NHC=cHC*MOLcylT, NCO2=cCO2*MOLcylT, NCO=cCO*MOLcylT, NO2=cO2*MOLcylT, NH2=cH2*MOLcylT, NH2O=cH2O*MOLcylT, NN2=cN2*MOLcylT}
      mask prompts: NHC "initial HC mol"; NCO2 "initial CO2 mol"; NCO "initial CO mol"; NO2 "initial O2 mol"; NH2 "initial H2 mol"; NH2O "initial H2O mol"; NN2 "initial N2 mol"
  mol_us : Outport  InitialOutput=0
  wires:
  Memory1/1 -> init&trig/2(value)
  trig_mix/1 -> Memory2/1
  Memory2/1 -> Mass_Int/2, init&trig/1(trig)
  add_fuel1/1(add_fuel) -> Sum/1
  Nfuel/1 -> add_fuel1/1(Nfuel)
  gas_in/1 -> add_fuel1/2(mol)
  init&trig/1(init) -> Mass_Int/3
  mix_mol/1 -> Memory1/1
  Mass_Int/1 -> mol_us/1
  burning/1 -> Sum/3
  Sum/1 -> Mass_Int/1
  gas_out/1 -> Sum/2

== system benchmark_model/ENGINE/engine_s/cylinders/cyl4/selectors/Triggered Subsystem1 ==
  sa : Inport
  Trigger : TriggerPort  VariantControl=(inherit)
  req_sa : Outport  InitialOutput=[20]
  wires:
  sa/1 -> req_sa/1

== system benchmark_model/ENGINE/engine_s/cylinders/cyl4/selectors/Triggered Subsystem2 ==
  int_mc : Inport
  Trigger : TriggerPort  VariantControl=(inherit)
  O2_mol : Outport  InitialOutput=[1.0e-19]
  wires:
  int_mc/1 -> O2_mol/1

== system benchmark_model/ENGINE/engine_s/cylinders/cyl4/selectors/Triggered Subsystem3 ==
  int_mc : Inport
  Trigger : TriggerPort  VariantControl=(inherit)
  MC : Outport  InitialOutput=[1.0e-19]
  wires:
  int_mc/1 -> MC/1

== system benchmark_model/ENGINE/engine_s/cylinders/cyl4/selectors/effective_O2_flow ==
  fml : Inport
  Gain : Gain  Gain=1+y/4
  Gain1 : Gain  Gain=0.5
  Gain2 : Gain  Gain=0.5
  Selector : Selector  InputPortWidth=7  IndexOptions=Index vector (dialog)  Indices=[4]  OutputSizes=1
  Selector1 : Selector  InputPortWidth=7  IndexOptions=Index vector (dialog)  Indices=[1]  OutputSizes=1
  Selector2 : Selector  InputPortWidth=7  IndexOptions=Index vector (dialog)  Indices=[3]  OutputSizes=1
  Selector3 : Selector  InputPortWidth=7  IndexOptions=Index vector (dialog)  Indices=[5]  OutputSizes=1
  Subtract : Sum  Inputs=+---
  fO2_mol : Outport
  wires:
  Gain2/1 -> Subtract/4
  Gain1/1 -> Subtract/3
  Selector3/1 -> Gain2/1
  Selector2/1 -> Gain1/1
  Gain/1 -> Subtract/2
  Selector1/1 -> Gain/1
  Selector/1 -> Subtract/1
  fml/1 -> Selector3/1, Selector2/1, Selector1/1, Selector/1
  Subtract/1 -> fO2_mol/1

== system benchmark_model/ENGINE/engine_s/cylinders/cyl4/selectors/fuel_behavior ==
  MC : Inport
  fi : Inport  Port=2
  rps : Inport  Port=3
  Trigger : TriggerPort  VariantControl=(inherit)
  Discrete-Time Integrator : DiscreteIntegrator  SampleTime=-1  ICPrevOutput=DiscIntNeverNeededParam  ICPrevScaledInput=DiscIntNeverNeededParam
  Terminator : Terminator
  Terminator3 : Terminator
  fc : Outport  InitialOutput=[0]
  sum_fc : Outport  Port=2  InitialOutput=[0]
  wires:
  Discrete-Time Integrator/1 -> sum_fc/1
  rps/1 -> Terminator/1
  MC/1 -> Terminator3/1
  fi/1 -> fc/1, Discrete-Time Integrator/1

== system benchmark_model/ENGINE/engine_s/cylinders/cyl4/selectors/selector ==
  st : Inport
  ECU_sa : Inport  Port=2
  ECU_fi : Inport  Port=3
  Saturation : Saturate  UpperLimit=inf  LowerLimit=0
  Selector : Selector  InputPortWidth=4  IndexOptions=Index vector (dialog)  Indices=[4]  OutputSizes=[(-2)]
  Selector2 : Selector  InputPortWidth=4  IndexOptions=Index vector (dialog)  Indices=[4]  OutputSizes=[(-2)]
  mod720(u,4*pi) : Subsystem
  rad : Outport
  sa : Outport  Port=2
  fi : Outport  Port=3
  wires:
  Selector2/1 -> sa/1
  ECU_fi/1 -> Saturation/1
  ECU_sa/1 -> Selector2/1
  st/1 -> Selector/1
  mod720(u,4*pi)/1(y) -> rad/1
  Saturation/1 -> fi/1
  Selector/1 -> mod720(u,4*pi)/1(u)

== system benchmark_model/ENGINE/engine_s/cylinders/cyl4/selectors/trig_MC ==
  deg : Inport
  ECU_vvt : Inport  Port=2
  Constant : Constant  Value=541+INC
  Gain : Gain  Gain=180/pi
  Relational Operator : RelationalOperator  OutDataTypeStr=boolean  RndMeth=Nearest
  Subtract : Sum
  flg_inc : Outport
  wires:
  Gain/1 -> Subtract/1
  Constant/1 -> Subtract/2
  ECU_vvt/1 -> Gain/1
  Subtract/1 -> Relational Operator/2
  Relational Operator/1 -> flg_inc/1
  deg/1 -> Relational Operator/1

== system benchmark_model/ENGINE/engine_s/cylinders/cyl4/selectors/trig_fi ==
  deg : Inport
  Constant : Constant  Value=361
  Relational Operator : RelationalOperator  OutDataTypeStr=boolean  RndMeth=Nearest
  flg_fi : Outport
  wires:
  Relational Operator/1 -> flg_fi/1
  deg/1 -> Relational Operator/1
  Constant/1 -> Relational Operator/2

== system benchmark_model/ENGINE/engine_s/cylinders/cyl4/selectors/trig_fi1 ==
  deg : Inport
  ECU_vvt : Inport  Port=2
  Constant : Constant  Value=360-INO-1
  Gain : Gain  Gain=180/pi
  Relational Operator : RelationalOperator  OutDataTypeStr=boolean  RndMeth=Nearest
  Subtract : Sum
  flg_fi : Outport
  wires:
  Constant/1 -> Subtract/2
  Subtract/1 -> Relational Operator/2
  Gain/1 -> Subtract/1
  ECU_vvt/1 -> Gain/1
  deg/1 -> Relational Operator/1
  Relational Operator/1 -> flg_fi/1

== system benchmark_model/ENGINE/engine_s/ex_chamber/In_vol/cal_cyl_state/cal_state ==
  m : Inport
  n : Inport  Port=2
  f : Inport  Port=3
  E : Inport  Port=4
  vol : Inport  Port=5
  Fcn : Fcn  Expr=2/u(1)*u(3)/u(2)
  Fcn1 : Fcn  Expr=2/u(1)*u(2)/(u(3)*Rabs)
  Mux : Mux  Inputs=3
  Mux1 : Mux
  Mux2 : Mux  Inputs=3
  Product1 : Product  Inputs=/*  RndMeth=Zero
  Product2 : Product  Inputs=*/  RndMeth=Zero
  Product3 : Product  Inputs=*/  RndMeth=Zero
  ex_st : Outport  PortDimensions=4  InitialOutput=0
  ex_temp : Outport  Port=2  InitialOutput=0
  wires:
  Fcn1/1 -> ex_temp/1
  Mux2/1 -> Fcn1/1
  E/1 -> Mux2/2, Mux/3
  f/1 -> Product1/2
  n/1 -> Mux2/3, Product1/1, Product2/2
  m/1 -> Product3/1, Product2/1
  Product3/1 -> Mux1/1  "dens"
  Product2/1 -> Mux1/3  "gas_c"
  Product1/1 -> Mux2/1, Mux/1, Mux1/4  "deg of freedom"
  vol/1 -> Product3/2, Mux/2
  Mux1/1 -> ex_st/1
  Mux/1 -> Fcn/1
  Fcn/1 -> Mux1/2  "pres"

== system benchmark_model/ENGINE/engine_s/in_chamber/In_vol/Mol_Int/signiture_EGR ==
  In : Inport
  Add : Sum  Inputs=+++
  Demux : Demux  Outputs=7
  Mux : Mux  Inputs=8
  Saturation : Saturate  UpperLimit=inf  LowerLimit=0
  Out : Outport
  wires:
  Mux/1 -> Out/1
  In/1 -> Demux/1
  Demux/1 -> Add/1, Mux/1
  Demux/2 -> Add/2, Mux/2
  Demux/3 -> Add/3, Mux/3
  Demux/4 -> Mux/4
  Demux/5 -> Mux/5
  Demux/6 -> Mux/6
  Demux/7 -> Mux/7
  Add/1 -> Saturation/1
  Saturation/1 -> Mux/8

== system benchmark_model/ENGINE/engine_s/in_chamber/In_vol/Mol_Int/signiture_EGR1 ==
  In : Inport
  Constant : Constant  Value=0
  Demux : Demux  Outputs=7
  Mux : Mux  Inputs=8
  Out : Outport
  wires:
  Demux/7 -> Mux/7
  Demux/6 -> Mux/6
  Demux/5 -> Mux/5
  Demux/4 -> Mux/4
  Demux/3 -> Mux/3
  Demux/2 -> Mux/2
  Demux/1 -> Mux/1
  In/1 -> Demux/1
  Mux/1 -> Out/1
  Constant/1 -> Mux/8

== system benchmark_model/ENGINE/engine_s/in_chamber/In_vol/Mol_Int/signiture_EGR2 ==
  In : Inport
  C_signed_C : Inport  Port=2
  Demux : Demux  Outputs=7
  Mux : Mux  Inputs=8
  Product : Product
  Saturation : Saturate  UpperLimit=inf  LowerLimit=0
  Sum of Elements : Sum  Inputs=+
  Out : Outport
  wires:
  Mux/1 -> Out/1
  In/1 -> Sum of Elements/1, Demux/1
  Demux/1 -> Mux/1
  Demux/2 -> Mux/2
  Demux/3 -> Mux/3
  Demux/4 -> Mux/4
  Demux/5 -> Mux/5
  Demux/6 -> Mux/6
  Demux/7 -> Mux/7
  Saturation/1 -> Mux/8
  Product/1 -> Saturation/1
  Sum of Elements/1 -> Product/1
  C_signed_C/1 -> Product/2

== system benchmark_model/ENGINE/engine_s/in_chamber/In_vol/Mol_Int/signiture_EGR3 ==
  In : Inport
  Demux : Demux  Outputs=8
  Mux : Mux  Inputs=7
  Out : Outport
  signed_C : Outport  Port=2
  wires:
  Mux/1 -> Out/1
  In/1 -> Demux/1
  Demux/1 -> Mux/1
  Demux/2 -> Mux/2
  Demux/3 -> Mux/3
  Demux/4 -> Mux/4
  Demux/5 -> Mux/5
  Demux/6 -> Mux/6
  Demux/7 -> Mux/7
  Demux/8 -> signed_C/1

== system benchmark_model/ENGINE/engine_s/in_chamber/In_vol/Mol_Int/signiture_EGR4 ==
  In : Inport
  Demux : Demux  Outputs=7
  Mux : Mux  Inputs=3
  Sum of Elements : Sum  Inputs=+
  Terminator{,1..3} (4 alike) : Terminator
  Out : Outport
  wires:
  Demux/3 -> Mux/3
  Demux/2 -> Mux/2
  Demux/1 -> Mux/1
  In/1 -> Demux/1
  Mux/1 -> Sum of Elements/1
  Demux/4 -> Terminator/1
  Demux/5 -> Terminator1/1
  Demux/6 -> Terminator2/1
  Demux/7 -> Terminator3/1
  Sum of Elements/1 -> Out/1

== system benchmark_model/ENGINE/engine_s/in_chamber/In_vol/cal_cyl_state/cal_state ==
  m : Inport
  n : Inport  Port=2
  f : Inport  Port=3
  E : Inport  Port=4
  vol : Inport  Port=5
  Fcn : Fcn  Expr=2/u(1)*u(3)/u(2)
  Mux : Mux  Inputs=3
  Mux1 : Mux
  Product1 : Product  Inputs=/*  RndMeth=Zero
  Product2 : Product  Inputs=*/  RndMeth=Zero
  Product3 : Product  Inputs=*/  RndMeth=Zero
  cyl_st : Outport  InitialOutput=0
  wires:
  Fcn/1 -> Mux1/2  "pres"
  Mux/1 -> Fcn/1
  Mux1/1 -> cyl_st/1
  vol/1 -> Mux/2, Product3/2
  Product1/1 -> Mux1/4, Mux/1  "deg of freedom"
  Product2/1 -> Mux1/3  "gas_c"
  Product3/1 -> Mux1/1  "dens"
  m/1 -> Product2/1, Product3/1
  n/1 -> Product1/1, Product2/2
  f/1 -> Product1/2
  E/1 -> Mux/3

== system benchmark_model/ENGINE/engine_s/cylinders/cyl1/cyl/Energy_Int/dvol ==
  rad : Inport
  rps : Inport  Port=2
  Product : Product  RndMeth=Zero
  func_d_cylvol(u,SPEC) : Subsystem
  dvol : Outport
  wires:
  rps/1 -> Product/2
  Product/1 -> dvol/1
  rad/1 -> func_d_cylvol(u,SPEC)/1(In1)
  func_d_cylvol(u,SPEC)/1(Out1) -> Product/1

== system benchmark_model/ENGINE/engine_s/cylinders/cyl1/cyl/cal_cyl_state/cal_state ==
  m : Inport
  n : Inport  Port=2
  f : Inport  Port=3
  E : Inport  Port=4
  vol : Inport  Port=5
  Fcn : Fcn  Expr=2/u[1]*u[3]/u[2]
  Fcn1 : Fcn  Expr=u[3]/u[1]/(Rabs/u[2])
  Mux : Mux  Inputs=3
  Mux1 : Mux
  Mux2 : Mux  Inputs=3
  Product1 : Product  Inputs=/*  RndMeth=Zero
  Product2 : Product  Inputs=*/  RndMeth=Zero
  Product3 : Product  Inputs=*/  RndMeth=Zero
  pc : Outport  InitialOutput=0
  tc : Outport  Port=2  InitialOutput=0
  cyl_st : Outport  Port=3  InitialOutput=0
  wires:
  Fcn/1 -> Mux1/2, Mux2/3, pc/1  "pres"
  Mux/1 -> Fcn/1
  Mux1/1 -> cyl_st/1
  vol/1 -> Mux/2, Product3/2
  Product1/1 -> Mux/1, Mux1/4  "deg of freedom"
  Product2/1 -> Mux2/2, Mux1/3  "gas_c"
  Product3/1 -> Mux2/1, Mux1/1  "dens"
  Mux2/1 -> Fcn1/1
  m/1 -> Product2/1, Product3/1
  n/1 -> Product1/1, Product2/2
  f/1 -> Product1/2
  E/1 -> Mux/3
  Fcn1/1 -> tc/1

== system benchmark_model/ENGINE/engine_s/cylinders/cyl1/cyl/crank/Subsystem1 ==
  trig_inj : Inport
  fc : Inport  Port=2
  N/s : Inport  Port=3
  Gain : Gain  Gain=MHC
  Integrator : Integrator  ExternalReset=rising
  Product : Product
  Relational Operator1 : RelationalOperator  OutDataTypeStr=boolean  RndMeth=Nearest
  N_fuel : Outport
  wires:
  trig_inj/1 -> Integrator/2
  Product/1 -> N_fuel/1
  Integrator/1 -> Relational Operator1/2
  Relational Operator1/1 -> Product/1
  fc/1 -> Relational Operator1/1
  N/s/1 -> Product/2, Gain/1
  Gain/1 -> Integrator/1

== system benchmark_model/ENGINE/engine_s/cylinders/cyl1/cyl/crank/inj_start ==
  rad : Inport
  Constant3 : Constant  Value=(360-INO+1)*pi/180
  Relational Operator2 : RelationalOperator  OutDataTypeStr=boolean  RndMeth=Nearest
  trig_inj : Outport
  wires:
  Constant3/1 -> Relational Operator2/2
  rad/1 -> Relational Operator2/1
  Relational Operator2/1 -> trig_inj/1

== system benchmark_model/ENGINE/engine_s/cylinders/cyl1/cyl/crank/mol_flow_rate ==
  rps : Inport
  Constant1 : Constant  Value=0.50*pi
  Constant2 : Constant  Value=MHC
  Divide2 : Product  Inputs=*/
  Divide3 : Product  Inputs=*/
  Divide4 : Product  Inputs=*/
  inje/s : Constant  Value=(DEN0*VH/14.5)
  N/s : Outport
  wires:
  Constant2/1 -> Divide3/2
  Divide3/1 -> N/s/1
  inje/s/1 -> Divide2/1
  Constant1/1 -> Divide4/1
  rps/1 -> Divide4/2
  Divide4/1 -> Divide2/2
  Divide2/1 -> Divide3/1

== system benchmark_model/ENGINE/engine_s/cylinders/cyl1/cyl/frame/Init_cyl_gas ==
  tr_inc : Inport
  mol_s : Inport  Port=2
  capture_cyl_state : Subsystem  TreatAsAtomicUnit=on
  init_gas : Outport
  Qmax : Outport  Port=2
  b_comp : Outport  Port=3
  af : Outport  Port=4
  wires:
  capture_cyl_state/3(init_gas) -> init_gas/1
  capture_cyl_state/2(b_comp) -> b_comp/1
  mol_s/1 -> capture_cyl_state/1(cyl_gas)
  capture_cyl_state/1(Qmax) -> Qmax/1
  capture_cyl_state/4(af) -> af/1
  tr_inc/1 -> capture_cyl_state/Trigger

== system benchmark_model/ENGINE/engine_s/cylinders/cyl1/cyl/frame/ratio_burnt1 ==
  rps : Inport
  rad : Inport  Port=2
  AF : Inport  Port=3
  KL : Inport  Port=4
  SA : Inport  Port=5
  EGR : Inport  Port=6
  VT : Inport  Port=7
  Add : Sum
  Constant : Constant  Value=(180-EXO-1)*pi/180+pi
  Constant1 : Constant  Value=0
  Constant2 : Constant  Value=pi
  Constant3 : Constant  Value=0
  Product : Product  RndMeth=Zero
  Relational Operator : RelationalOperator  Operator=<  OutDataTypeStr=boolean  RndMeth=Nearest
  Switch : Switch  Threshold=0.5
  Switch1 : Switch  Threshold=0.5
  mod720(u,4*pi) : Subsystem
  murnt_ratio : Subsystem
  burnt_ratio : Outport  PortDimensions=1  InitialOutput=0
  QR : Outport  Port=2  PortDimensions=1  InitialOutput=0
  Q : Outport  Port=3  PortDimensions=1  InitialOutput=0
  wires:
  murnt_ratio/1(q) -> Switch/1
  mod720(u,4*pi)/1(y) -> murnt_ratio/1(u), Relational Operator/1
  rps/1 -> murnt_ratio/3(rps), Product/2
  AF/1 -> murnt_ratio/5(AF)
  KL/1 -> murnt_ratio/4(KL)
  SA/1 -> murnt_ratio/2(SA)
  Constant/1 -> Relational Operator/2
  Relational Operator/1 -> Switch1/2, Switch/2
  Constant1/1 -> Switch/3
  Switch/1 -> Product/1, QR/1
  Product/1 -> burnt_ratio/1
  EGR/1 -> murnt_ratio/6(EGR)
  Add/1 -> mod720(u,4*pi)/1(u)
  rad/1 -> Add/2
  Constant2/1 -> Add/1
  murnt_ratio/2(Q) -> Switch1/1
  Constant3/1 -> Switch1/3
  Switch1/1 -> Q/1
  VT/1 -> murnt_ratio/7(VT)

== system benchmark_model/ENGINE/engine_s/cylinders/cyl1/cyl/heat_trans/cal_cyl_ar ==
  vol : Inport
  Add2 : Sum
  Constant1 : Constant  Value=2*pi*BORE
  Constant2 : Constant  Value=AREA
  Gain1 : Gain  Gain=2
  Product1 : Product  Inputs=*/  RndMeth=Zero
  Product2 : Product  RndMeth=Zero
  cyl_ar : Outport
  wires:
  Constant2/1 -> Product1/2, Gain1/1
  Gain1/1 -> Add2/2
  vol/1 -> Product1/1
  Add2/1 -> cyl_ar/1
  Product1/1 -> Product2/2
  Constant1/1 -> Product2/1
  Product2/1 -> Add2/1

== system benchmark_model/ENGINE/engine_s/cylinders/cyl1/cyl/heat_trans/cal_qw ==
  pc : Inport
  rps : Inport  Port=2
  Tg : Inport  Port=3
  Tw : Inport  Port=4
  Fcn : Fcn  Expr=(u(1)*u(2))^0.786*u(3)^(-0.525)*(u(3)-u(4))
  Mux3 : Mux
  Saturation : Saturate  UpperLimit=inf  LowerLimit=1.0e-16
  qw : Outport
  wires:
  Mux3/1 -> Saturation/1
  Fcn/1 -> qw/1
  Tw/1 -> Mux3/4
  pc/1 -> Mux3/1
  rps/1 -> Mux3/2
  Tg/1 -> Mux3/3
  Saturation/1 -> Fcn/1
